simulink model "HW2P5"  (R2020b)
settings: Solver=VariableStepAuto  StartTime=0.0  StopTime=10.0  RelTol=1e-3
values from neighbouring files (symbols this model uses):
  n = 0 : 120    [HW1.m]
undefined symbols (not defined in the file or in its folder): m
settings Model: Creator=mluser  LastModifiedBy=mluser

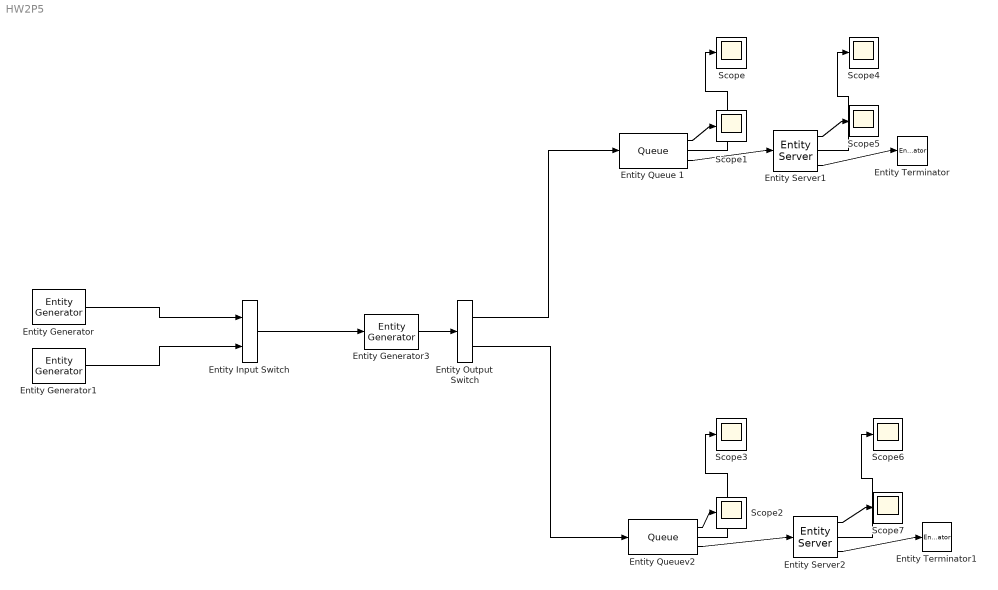
== system HW2P5 ==
  Entity Input Switch : EntityInputSwitch  InputPortMessageModes=m,m  OutputPortMessageModes=m
  Entity Output Switch : EntityOutputSwitch  InputPortMessageModes=m  OutputPortMessageModes=m,m  SwitchingCriterion=From attribute  SwitchAttributeName=Attribute1
  Entity Generator : EntityGenerator  OutputPortMessageModes=m  Period=0.11111  EntityType=Structured  EntityTypeName=Entity1
  Entity Generator1 : EntityGenerator  OutputPortMessageModes=m  Period=0.33333  EntityType=Structured  EntityTypeName=Entity1
  Entity Generator3 : EntityGenerator  InputPortMessageModes=m  OutputPortMessageModes=m  GenerationMethod=Event-based  Period=0.11111  GenerateAction=|  EntityType=Structured  EntityTypeName=Entity3
      | rnum = rand();
      | 
      | if rnum > 0.75
      |     entity.Attribute1 = 1; %75 percent
      | elseif rnum > 0.25
      |     entity.Attribute1 = 2; %25 percent
      | end
      settings: InputPortMap=u0
  Entity Queue 1 : Queue  InputPortMessageModes=m  OutputPortMessageModes=n,n,m  AverageWait=on  AverageQueueLength=on
      settings: OutputPortMap=o2,o3,o5
  Entity Queuev2 : Queue  InputPortMessageModes=m  OutputPortMessageModes=n,n,m  AverageWait=on  AverageQueueLength=on
      settings: OutputPortMap=o2,o3,o5
  Entity Server1 : EntityServer  InputPortMessageModes=m  OutputPortMessageModes=n,n,m  Capacity=1  ServiceTimeValue=0.071429  AverageWait=on  Utilization=on
      settings: OutputPortMap=o4,o5,o9
  Entity Server2 : EntityServer  InputPortMessageModes=m  OutputPortMessageModes=n,n,m  Capacity=1  ServiceTimeValue=0.08333  AverageWait=on  Utilization=on
      settings: OutputPortMap=o4,o5,o9
  Entity Terminator : EntityTerminator  InputPortMessageModes=m
  Entity Terminator1 : EntityTerminator  InputPortMessageModes=m
  Scope{,1..7} (8 alike) : Scope
  wires:
  Entity Queue 1/3 -> Entity Server1/1
  Entity Queuev2/3 -> Entity Server2/1
  Entity Server1/3 -> Entity Terminator/1
  Entity Server2/3 -> Entity Terminator1/1
  Entity Queue 1/1 -> Scope1/1
  Entity Queuev2/1 -> Scope2/1
  Entity Queuev2/2 -> Scope3/1
  Entity Queue 1/2 -> Scope/1
  Entity Output Switch/1 -> Entity Queue 1/1
  Entity Output Switch/2 -> Entity Queuev2/1
  Entity Generator3/1 -> Entity Output Switch/1
  Entity Generator/1 -> Entity Input Switch/1
  Entity Generator1/1 -> Entity Input Switch/2
  Entity Input Switch/1 -> Entity Generator3/1
  Entity Server1/2 -> Scope4/1
  Entity Server1/1 -> Scope5/1
  Entity Server2/2 -> Scope6/1
  Entity Server2/1 -> Scope7/1
